simulink model "rjsh"  (Simulink 3.00)
settings: Solver=ode45  StartTime=0.0  StopTime=30  MaxStep=0.01  RelTol=1e-3  AbsTol=1e-3
undefined symbols (not defined in the file or in its folder): offset
settings Model: SaveTime=off  SaveOutput=off

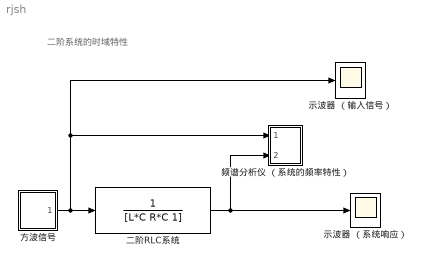
== system rjsh ==
  note: 二阶系统的时域特性
  二阶RLC系统 : TransferFcn  Numerator=[1]  Denominator=[L*C R*C 1]  mask( 单元7){@1=2, @2=1, @3=0.01}
      mask prompts: @1 "电阻值（欧）："; @2 "电感值（亨）："; @3 "电容值（法）："
      mask help: 单元7
      mask init:
      | R=@1;L=@2;C=@3;
      mask Display: plot([3 5 5 5],[2 2 1.5 2.5],[5 9],[2.5 2.5],[5 9],[1.5 1.5],[9 9],[2.5 1.5],[9 11],[2 2],[11:1/7:12],[2 2.5 2.707 2.866 2.866 2.707 2.5 2],[12:1/7:13],[2 2.5 2.707 2.866 2.866 2.707 2.5 2],[13:1/7:14],[2 2.5 2.707 2.866 2.866 2.707 2.5 2],[14:1/7:15],[2 2.5 2.707 2.866 2.866 2.707 2.5 2],[15 21],[2 2],[18 18 16 20],[2 0 0 0],[16 20],[-1 -1],[18 18 17 19],[-1 -3 -3 -3]);
  方波信号 : Subsystem  mask(Pulse Generator){@1=20, @2=20, @3=1, @4=1}
      mask prompts: @1 "Pulse period (secs):"; @2 "Pulse width:"; @3 "Pulse height:"; @4 "Pulse start time:"
      mask help: Pulse Generator.
      mask init:
      | Ts=@1; du=@2; ht=@3; stt=@4; ini=ones(length(ht),1); st1=rem(stt,Ts); st2=rem(stt+du,Ts);if(Ts<=1.2*du),ini=zeros(length(ht),1);end;
      mask Help: Pulse generator which ensures pulse\ntransitions are hit. Provides a vector of pulses when the height is entered as a vector.\nUnmask to see how it works.
      mask Display: plot(0,0,100,100,[90,75,75,60,60,35,35,20,20,10],[20,20,80,80,20,20,80,80,20,20])
  频谱分析仪 （系统的频率特性） : Subsystem  mask(Spectrum analyzer.){@1=512, @2=1024, @3=100, @4=0.05}
      mask prompts: @1 "Length of buffer:"; @2 "Number of points for fft:"; @3 "Plot after how many points:"; @4 "Sample time:"
      mask help:
      | Spectrum analyser using graph window.
      | Hook input 1 to system input.
      | Hook input 2 to system output.
      mask init:
      | npts=@1; fftpts=@2; HowOften=@3; ts=@4(1); if length(@4) > 1, offset = @4(2), else, offset = 0; end
      mask Help: Hook the system's input to the first port of this block and the system's output to second port. Results are displayed as the frequency response of this system. Use signals with high harmonic content for best results.
      mask Display: plot(0,0,100,100,[11,93,93,11,11],[90,90,40,40,90],[90,80,72,64,55,45,41,36,20],[50,50,52,59,67,75,78,80,80])
  "示波器 （输入信号） " : Scope
      settings: TimeRange=30.000000  YMin=-1.5  YMax=1.5  SaveToWorkspace=off  SaveName=ScopeData  DataFormat=Matrix
  示波器 （系统响应） : Scope
      settings: TimeRange=30.000000  YMin=-1.5  YMax=1.5  SaveToWorkspace=off  SaveName=ScopeData  DataFormat=Matrix
  wires:
  方波信号/1(out_1) -> 二阶RLC系统/1, "示波器 （输入信号） "/1, 频谱分析仪 （系统的频率特性）/1(system input)
  二阶RLC系统/1 -> 示波器 （系统响应）/1, 频谱分析仪 （系统的频率特性）/2(system output)

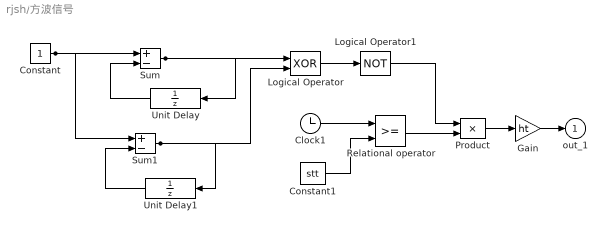
== system rjsh/方波信号 ==
  Clock1 : Clock
      settings: DisplayTime=off  Decimation=10
  Constant : Constant  Value=1
  Constant1 : Constant  Value=stt
  Gain : Gain  Gain=ht  SaturateOnIntegerOverflow=on
  Logical Operator : Logic  Operator=XOR  Inputs=2
  Logical Operator1 : Logic  Operator=NOT  Inputs=1
  Product : Product  Inputs=2  SaturateOnIntegerOverflow=on
  Relational operator : RelationalOperator  Operator=>=
  Sum : Sum  Inputs=+-  SaturateOnIntegerOverflow=on
  Sum1 : Sum  Inputs=+-  SaturateOnIntegerOverflow=on
  Unit Delay : UnitDelay  Orientation=left  X0=0  SampleTime=[Ts,st1]
  Unit Delay1 : UnitDelay  Orientation=left  X0=ini  SampleTime=[Ts,st2]
  out_1 : Outport  Port=1
  wires:
  Unit Delay1/1 -> Sum1/2
  Sum1/1 -> Logical Operator/2, Unit Delay1/1
  Constant/1 -> Sum1/1, Sum/1
  Sum/1 -> Logical Operator/1, Unit Delay/1
  Unit Delay/1 -> Sum/2
  Clock1/1 -> Relational operator/1
  Relational operator/1 -> Product/2
  Product/1 -> Gain/1
  Gain/1 -> out_1/1
  Constant1/1 -> Relational operator/2
  Logical Operator/1 -> Logical Operator1/1
  Logical Operator1/1 -> Product/1

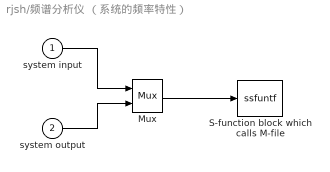
== system rjsh/频谱分析仪 （系统的频率特性） ==
  system input : Inport  Port=1  PortWidth=-1  SampleTime=-1  DataType=auto
      settings: SignalType=auto
  system output : Inport  Port=2  PortWidth=-1  SampleTime=-1  DataType=auto
      settings: SignalType=auto
  Mux : Mux  Inputs=2
      settings: DisplayOption=none
  S-function block which calls M-file : S-Function  FunctionName=ssfuntf  Parameters=fftpts,npts,HowOften,offset,ts,0  PortCounts=[]  SFunctionModules=''
  wires:
  system output/1 -> Mux/2
  system input/1 -> Mux/1
  Mux/1 -> S-function block which calls M-file/1
